simulink model "induction_machine"  (Simulink 6.3)
settings: Solver=ode45  StartTime=0.0  StopTime=10.0  RelTol=1e-3
libraries: powerlib x4
settings Model: LastModifiedBy=Administrator

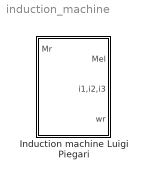
== system induction_machine ==
  Induction machine Luigi Piegari : Subsystem  mask{Lm=0.151, Lr=0.1513, Ls=0.1513, rs=0.03552, rr=0.02092, p=2, J=2.5}

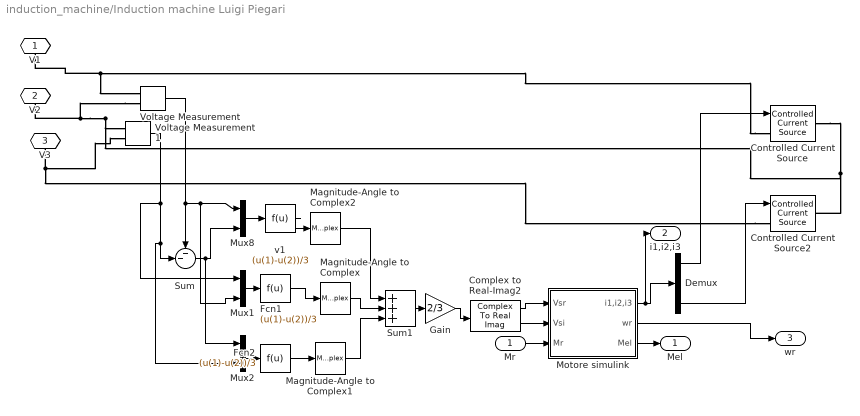
== system induction_machine/Induction machine Luigi Piegari ==
  Mr : Inport
  Complex to Real-Imag2 : ComplexToRealImag
  Controlled Current Source : powerlib/Electrical Sources/Controlled Current Source  Initialize=off  Amplitude=0  Phase=0  Frequency=0  Measurements=None
  Controlled Current Source2 : powerlib/Electrical Sources/Controlled Current Source  Initialize=off  Amplitude=0  Phase=0  Frequency=0  Measurements=None
  Demux : Demux  Outputs=3
  Fcn1 : Fcn  Expr=(u(1)-u(2))/3
  Fcn2 : Fcn  Expr=(u(1)-u(2))/3
  Gain : Gain  Gain=2/3
  Magnitude-Angle to Complex : MagnitudeAngleToComplex  Input=Magnitude  ConstantPart=2*pi/3
  Magnitude-Angle to Complex1 : MagnitudeAngleToComplex  Input=Magnitude  ConstantPart=4*pi/3
  Magnitude-Angle to Complex2 : MagnitudeAngleToComplex  Input=Magnitude
  Motore simulink : Subsystem
  Mux1 : Mux  Inputs=2
  Mux2 : Mux  Inputs=2
  Mux8 : Mux  Inputs=2
  Sum : Sum  Inputs=--|
  Sum1 : Sum  Inputs=+++
  Voltage Measurement : powerlib/Measurements/Voltage Measurement  PhasorSimulation=off  OutputType=Complex  PSBequivalent=0
  Voltage Measurement1 : powerlib/Measurements/Voltage Measurement  PhasorSimulation=off  OutputType=Complex  PSBequivalent=0
  v1 : Fcn  Expr=(u(1)-u(2))/3
  V1 : PMIOPort  Orientation=down  Port=1  Side=Left
  V2 : PMIOPort  Orientation=down  Port=2  Side=Left
  V3 : PMIOPort  Orientation=down  Port=3  Side=Left
  Mel : Outport
  i1,i2,i3 : Outport  Port=2
  wr : Outport  Port=3
  wires:
  Complex to Real-Imag2/1 -> Motore simulink/1(Vsr)
  Complex to Real-Imag2/2 -> Motore simulink/2(Vsi)
  Motore simulink/2(wr) -> wr/1
  Motore simulink/1(i1,i2,i3) -> Demux/1, i1,i2,i3/1
  Demux/1 -> Controlled Current Source/1
  Demux/3 -> Controlled Current Source2/1
  Voltage Measurement/1 -> Sum/1, Mux8/1, Mux1/2
  Voltage Measurement1/1 -> Mux1/1, Sum/2, Mux2/2
  Sum/1 -> Mux8/2, Mux2/1
  Mux8/1 -> v1/1
  Mux1/1 -> Fcn1/1
  Mux2/1 -> Fcn2/1
  Fcn1/1 -> Magnitude-Angle to Complex/1
  Fcn2/1 -> Magnitude-Angle to Complex1/1
  Magnitude-Angle to Complex/1 -> Sum1/2
  Magnitude-Angle to Complex1/1 -> Sum1/3
  v1/1 -> Magnitude-Angle to Complex2/1
  Magnitude-Angle to Complex2/1 -> Sum1/1
  Mr/1 -> Motore simulink/3(Mr)
  Motore simulink/3(Mel) -> Mel/1
  Sum1/1 -> Gain/1
  Gain/1 -> Complex to Real-Imag2/1
  connections:
  Controlled Current Source/LConn1 -- V1/RConn1 -- Voltage Measurement/LConn1
  Controlled Current Source2/LConn1 -- Voltage Measurement1/LConn2 -- V3/RConn1
  Voltage Measurement/LConn2 -- V2/RConn1 -- Controlled Current Source/RConn1 -- Controlled Current Source2/RConn1 -- Voltage Measurement1/LConn1

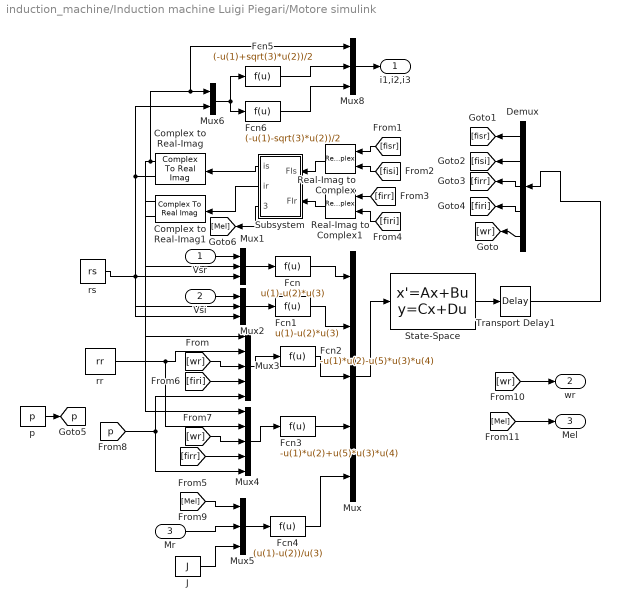
== system induction_machine/Induction machine Luigi Piegari/Motore simulink ==
  Vsr : Inport
  Vsi : Inport  Port=2
  Mr : Inport  Port=3
  Complex to Real-Imag : ComplexToRealImag  Orientation=left
  Complex to Real-Imag1 : ComplexToRealImag  Orientation=left
  Demux : Demux  Orientation=left  Outputs=5
  Fcn : Fcn  Expr=u(1)-u(2)*u(3)
  Fcn1 : Fcn  Expr=u(1)-u(2)*u(3)
  Fcn2 : Fcn  Expr=-u(1)*u(2)-u(5)*u(3)*u(4)
  Fcn3 : Fcn  Expr=-u(1)*u(2)+u(5)*u(3)*u(4)
  Fcn4 : Fcn  Expr=(u(1)-u(2))/u(3)
  Fcn5 : Fcn  Expr=(-u(1)+sqrt(3)*u(2))/2
  Fcn6 : Fcn  Expr=(-u(1)-sqrt(3)*u(2))/2
  J : Constant  Value=J
  Mux : Mux  Inputs=5
  Mux{1..2,5,8} (4 alike) : Mux  Inputs=3
  Mux3 : Mux  Inputs=5
  Mux4 : Mux  Inputs=5
  Mux6 : Mux  Inputs=2
  Real-Imag to Complex : RealImagToComplex  Orientation=left
  Real-Imag to Complex1 : RealImagToComplex  Orientation=left
  State-Space : StateSpace  A=[0 0 0 0 0; 0 0 0 0 0; 0 0 0 0 0; 0 0 0 0 0; 0 0 0 0 0]  B=[1 0 0 0 0; 0 1 0 0 0; 0 0 1 0 0; 0 0 0 1 0; 0 0 0 0 1]  C=[1 0 0 0 0; 0 1 0 0 0; 0 0 1 0 0; 0 0 0 1 0; 0 0 0 0 1]  D=[0 0 0 0 0; 0 0 0 0 0; 0 0 0 0 0; 0 0 0 0 0; 0 0 0 0 0]
  Subsystem : Subsystem  Orientation=left
  Transport Delay1 : TransportDelay  DelayTime=1e-5
  p : Constant  Value=p
  rr : Constant  Value=rr
  rs : Constant  Value=rs
  i1,i2,i3 : Outport
  wr : Outport  Port=2
  Mel : Outport  Port=3
  tag scope: p=global
  wires:
  State-Space/1 -> Transport Delay1/1
  Transport Delay1/1 -> Demux/1
  Mux/1 -> State-Space/1
  Real-Imag to Complex/1 -> Subsystem/1(FIs)
  Real-Imag to Complex1/1 -> Subsystem/2(FIr)
  Subsystem/1(is) -> Complex to Real-Imag/1
  Subsystem/2(ir) -> Complex to Real-Imag1/1
  Fcn/1 -> Mux/1
  Fcn1/1 -> Mux/2
  Fcn2/1 -> Mux/3
  Mux1/1 -> Fcn/1
  Mux2/1 -> Fcn1/1
  Mux3/1 -> Fcn2/1
  Complex to Real-Imag/1 -> Mux1/2, Mux6/1, Mux8/1
  Complex to Real-Imag/2 -> Mux2/2, Mux6/2
  Complex to Real-Imag1/1 -> Mux3/1
  rs/1 -> Mux1/3, Mux2/3
  rr/1 -> Mux3/2, Mux4/2
  Demux/5 -> [wr]
  [wr] -> Mux3/3
  Demux/1 -> [fisr]
  Demux/2 -> [fisi]
  Demux/3 -> [firr]
  Demux/4 -> [firi]
  [fisr] -> Real-Imag to Complex/1
  [fisi] -> Real-Imag to Complex/2
  [firr] -> Real-Imag to Complex1/1
  [firi] -> Real-Imag to Complex1/2
  [firi] -> Mux3/4
  [p] -> Mux3/5, Mux4/5
  Fcn3/1 -> Mux/4
  Mux4/1 -> Fcn3/1
  Complex to Real-Imag1/2 -> Mux4/1
  [wr] -> Mux4/3
  [firr] -> Mux4/4
  p/1 -> [p]
  Subsystem/3(Mel) -> [Mel]
  [Mel] -> Mux5/1
  Mr/1 -> Mux5/2
  J/1 -> Mux5/3
  Mux5/1 -> Fcn4/1
  Fcn4/1 -> Mux/5
  Mux6/1 -> Fcn5/1, Fcn6/1
  Mux8/1 -> i1,i2,i3/1
  Vsr/1 -> Mux1/1
  Vsi/1 -> Mux2/1
  [wr] -> wr/1
  [Mel] -> Mel/1
  Fcn5/1 -> Mux8/2
  Fcn6/1 -> Mux8/3

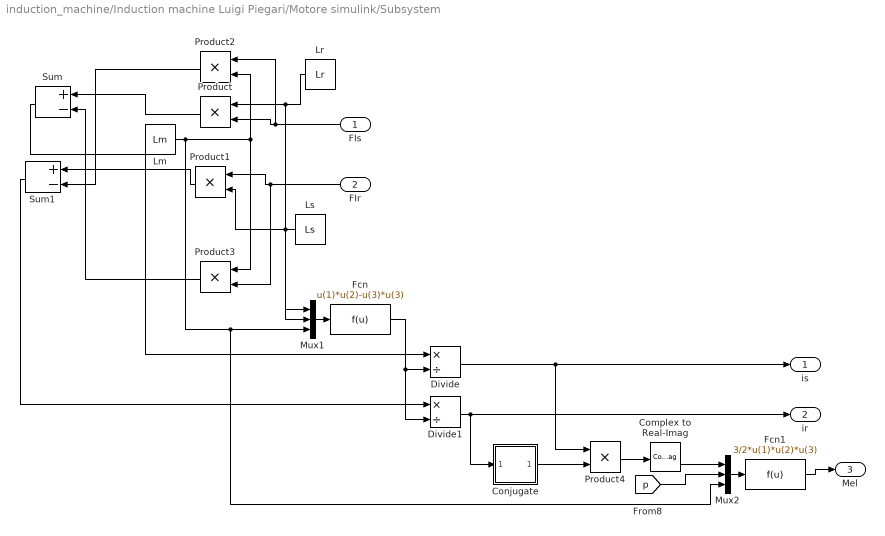
== system induction_machine/Induction machine Luigi Piegari/Motore simulink/Subsystem ==
  FIs : Inport  Orientation=left
  FIr : Inport  Orientation=left  Port=2
  Complex to Real-Imag : ComplexToRealImag
  Conjugate : Subsystem
  Divide : Product  Inputs=*/  OutScaling=2^-10
  Divide1 : Product  Inputs=*/  OutScaling=2^-10
  Fcn : Fcn  Expr=u(1)*u(2)-u(3)*u(3)
  Fcn1 : Fcn  Expr=3/2*u(1)*u(2)*u(3)
  Lm : Constant  Value=Lm
  Lr : Constant  Orientation=left  Value=Lr
  Ls : Constant  Orientation=left  Value=Ls
  Mux1 : Mux  Inputs=3
  Mux2 : Mux  Inputs=3
  Product{,1..3} (4 alike) : Product  Orientation=left  RndMeth=Zero
  Product4 : Product  RndMeth=Zero
  Sum : Sum  Orientation=left  Inputs=+-
  Sum1 : Sum  Orientation=left  Inputs=+-
  is : Outport
  ir : Outport  Port=2
  Mel : Outport  Port=3
  wires:
  Lr/1 -> Product/1, Mux1/2
  FIs/1 -> Product2/1, Product/2
  Ls/1 -> Product1/2, Mux1/1
  FIr/1 -> Product3/2, Product1/1
  Lm/1 -> Product2/2, Product3/1, Mux1/3, Mux2/3
  Product/1 -> Sum/1
  Product3/1 -> Sum/2
  Product1/1 -> Sum1/1
  Product2/1 -> Sum1/2
  Mux1/1 -> Fcn/1
  Fcn/1 -> Divide/2, Divide1/2
  Sum/1 -> Divide/1
  Sum1/1 -> Divide1/1
  Divide/1 -> is/1, Product4/1
  Divide1/1 -> ir/1, Conjugate/1(In1)
  Conjugate/1(Out1) -> Product4/2
  Product4/1 -> Complex to Real-Imag/1
  Mux2/1 -> Fcn1/1
  Complex to Real-Imag/2 -> Mux2/1
  [p] -> Mux2/2
  Fcn1/1 -> Mel/1

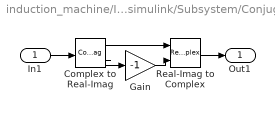
== system induction_machine/Induction machine Luigi Piegari/Motore simulink/Subsystem/Conjugate ==
  In1 : Inport
  Complex to Real-Imag : ComplexToRealImag
  Gain : Gain  Gain=-1
  Real-Imag to Complex : RealImagToComplex
  Out1 : Outport
  wires:
  Gain/1 -> Real-Imag to Complex/2
  Complex to Real-Imag/2 -> Gain/1
  Complex to Real-Imag/1 -> Real-Imag to Complex/1
  In1/1 -> Complex to Real-Imag/1
  Real-Imag to Complex/1 -> Out1/1
